simulink model "gm_sampleModel1739_2_sub"  (R2023a)
settings: Solver=VariableStepAuto  StartTime=0.0  StopTime=10.0  RelTol=1e-3
libraries: hdlsllib x2, simulink x1
settings Model: Creator=user1  LastModifiedBy=user1
settings OptimizationCC: BlockReduction=off  ConditionallyExecuteInputs=off
settings DebuggingCC: InheritedTsInSrcMsg=none

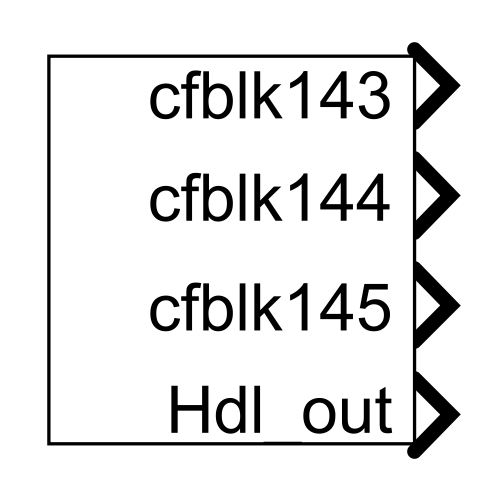
[thumbnail: Simulink's stored preview of the top-level diagram]
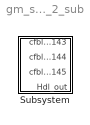
== system gm_sampleModel1739_2_sub ==
  Subsystem : Subsystem

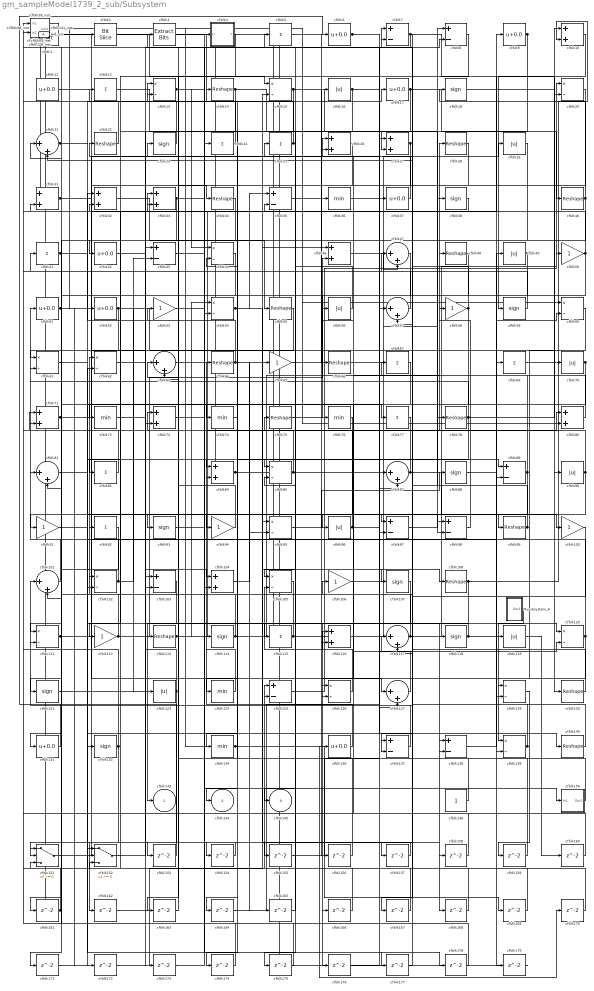
== system gm_sampleModel1739_2_sub/Subsystem ==
  Mysubsystem_6 : Subsystem
  cfblk1 : hdlsllib/Logic and Bit Operations/Bit Shift  mode=Shift Left Logical  N=0
  cfblk{10,26..27,31..33,46,71,73,80,84,104,116} (13 alike) : Sum  OutDataTypeStr=uint8
  cfblk{50,53,58,65,91,94,100,106,112} (9 alike) : Gain  OutDataTypeStr=uint8
  cfblk{21,47,57,63,81,87,101,117,127} (9 alike) : Sum  Inputs=|++  OutDataTypeStr=uint8
  cfblk{13,15,20,44,54,60..62,85,95,102,105,111,120,126,129,139} (17 alike) : Product  Inputs=*/  OutDataTypeStr=uint8  RndMeth=Zero  SaturateOnIntegerOverflow=on
  cfblk{7..8,35,43,89,97..98,103,125,137..138} (11 alike) : Sum  Inputs=+-  OutDataTypeStr=uint8
  cfblk{18,23,38,59,88,93,107,114,118,121,132} (11 alike) : Signum
  cfblk{14,22,28,34,40,48,55,64,66,75,78,99,108,113,130,140} (16 alike) : Reshape
  cfblk109_inst : Subsystem
  cfblk{6,9,11,17,37,42,51..52,131,136} (10 alike) : Bias  Bias=0.0  SaturateOnIntegerOverflow=off
  cfblk110_inst : Subsystem
  cfblk{5,12,24..25,41,67,69,77,82,92,115} (11 alike) : Sum  Inputs=+  OutDataTypeStr=uint8
  cfblk{16,29,49,56,70,90,96,119,123} (9 alike) : Abs  OutDataTypeStr=uint8  SaturateOnIntegerOverflow=off
  cfblk{36,72,74,76,124,134} (6 alike) : MinMax  OutDataTypeStr=uint8
  cfblk128_inst : Subsystem
  cfblk133_inst : Subsystem
  cfblk141_inst : Subsystem
  cfblk148 : Constant  OutDataTypeStr=uint8  SampleTime=-1
  cfblk150 : Subsystem
  cfblk151 : Switch  OutDataTypeStr=uint8  SaturateOnIntegerOverflow=off  InputSameDT=off
  cfblk152 : Switch  OutDataTypeStr=uint8  SaturateOnIntegerOverflow=off  InputSameDT=off
  cfblk{153..179} (27 alike) : Delay  SampleTime=1
  cfblk2 : hdlsllib/Logic and Bit Operations/Bit Slice  lidx=7  ridx=0
  cfblk3 : simulink/Logic and Bit Operations/Extract Bits  bitsToExtract=Upper half  numBits=8  bitIdxRange=[0 7]  outScalingMode=Preserve fixed-point scaling
      settings: LibrarySourceBlock=|
      | hdlsllib/Logic and Bit
      | Operations/Extract Bits
  cfblk39_inst : Subsystem
  cfblk4 : Subsystem  mask(Detect Rise Nonnegative){vinit=double(0), InputProcessing=Elements as channels (sample based), OutDataTypeStr=uint8}
      mask prompts: vinit "Simulink:masks:InitialCondition_MP"; InputProcessing "Simulink:masks:InputProcessing_MP"; OutDataTypeStr "Simulink:masks:OutputDataType_MP"
      mask help: Simulink:masks:DetectRiseNonnegative_MD
      mask init:
      | InputProcessing = 'Elements as channels (sample based)';
      | OutDataTypeStr = 'uint8';
      | vinit = double(0);
      mask TypeOptions InputProcessing: Simulink:masks:ColumnsAsChannelsFrameBased | Simulink:masks:ElementsAsChannelsSampleBased
      mask TypeOptions OutDataTypeStr: Simulink:masks:uint8 | Simulink:masks:boolean
      mask Display: fprintf('U >= 0\n&  NOT\nU/z >= 0')
  cfblk68_inst : Subsystem
  cfblk83_inst : Subsystem
  cfblk143 : Outport  OutDataTypeStr=uint8  SampleTime=1  VectorParamsAs1DForOutWhenUnconnected=off
  cfblk144 : Outport  Port=2  OutDataTypeStr=uint8  SampleTime=1  VectorParamsAs1DForOutWhenUnconnected=off
  cfblk145 : Outport  Port=3  OutDataTypeStr=uint8  SampleTime=1  VectorParamsAs1DForOutWhenUnconnected=off
  Hdl_out : Outport  Port=4  OutDataTypeStr=uint8  SampleTime=1
  wires:
  Mysubsystem_6/1(Out1) -> cfblk139/1
  cfblk1/1 -> cfblk34/1, cfblk127/1
  cfblk10/1 -> cfblk59/1
  cfblk100/1 -> cfblk125/1
  cfblk101/1 -> cfblk51/1
  cfblk102/1 -> cfblk81/1, cfblk43/2
  cfblk103/1 -> cfblk143/1
  cfblk104/1 -> cfblk65/1
  cfblk105/1 -> cfblk63/1
  cfblk106/1 -> cfblk29/1
  cfblk107/1 -> cfblk176/1
  cfblk108/1 -> cfblk10/2, cfblk168/1
  cfblk109_inst/1(out1) -> cfblk2/1
  cfblk11/1 -> cfblk77/1
  cfblk110_inst/1(out1) -> cfblk133_inst/2(in2), cfblk133_inst/1(in1), cfblk119/1
  cfblk111/1 -> cfblk35/2, cfblk23/1
  cfblk112/1 -> cfblk46/2, cfblk141_inst/1(in1)
  cfblk113/1 -> cfblk9/1, cfblk80/1, cfblk54/1
  cfblk114/1 -> cfblk71/2, cfblk28/1
  cfblk115/1 -> cfblk39_inst/1(in1), cfblk21/1
  cfblk116/1 -> cfblk48/1
  cfblk117/1 -> cfblk62/1, cfblk20/1
  cfblk118/1 -> cfblk113/1, cfblk60/2
  cfblk119/1 -> cfblk160/1
  cfblk12/1 -> cfblk98/1
  cfblk120/1 -> cfblk64/1, cfblk167/1, cfblk166/1
  cfblk121/1 -> cfblk103/2
  cfblk123/1 -> cfblk103/1, cfblk153/1
  cfblk124/1 -> cfblk84/2
  cfblk125/1 -> cfblk50/1
  cfblk126/1 -> cfblk105/2
  cfblk127/1 -> cfblk26/1
  cfblk128_inst/1(out1) -> cfblk87/1
  cfblk129/1 -> cfblk159/1
  cfblk13/1 -> cfblk54/2, cfblk44/1
  cfblk130/1 -> cfblk92/1
  cfblk131/1 -> cfblk6/1
  cfblk132/1 -> cfblk68_inst/1(in1), cfblk32/2, cfblk162/1
  cfblk133_inst/1(out1) -> cfblk60/1
  cfblk134/1 -> cfblk170/1, cfblk169/1
  cfblk136/1 -> cfblk114/1
  cfblk137/1 -> cfblk101/1
  cfblk138/1 -> cfblk69/1
  cfblk139/1 -> cfblk73/1, cfblk110_inst/2(in2), cfblk106/1
  cfblk14/1 -> cfblk63/2, cfblk27/2
  cfblk140/1 -> cfblk22/1
  cfblk141_inst/1(out1) -> cfblk31/1, cfblk136/1
  cfblk148/1 -> cfblk5/1
  cfblk15/1 -> cfblk78/1, cfblk73/2, cfblk57/1
  cfblk150/1(Out1) -> cfblk26/2
  cfblk151/1 -> cfblk49/1
  cfblk152/1 -> cfblk7/1
  cfblk153/1 -> cfblk109_inst/2(in2)
  cfblk154/1 -> cfblk152/2
  cfblk155/1 -> cfblk87/2
  cfblk156/1 -> cfblk44/2
  cfblk157/1 -> cfblk151/2
  cfblk158/1 -> cfblk83_inst/2(in2)
  cfblk159/1 -> cfblk13/1
  cfblk16/1 -> cfblk37/1, cfblk174/1
  cfblk160/1 -> cfblk116/1
  cfblk161/1 -> cfblk39_inst/2(in2), Hdl_out/1
  cfblk162/1 -> cfblk15/2
  cfblk163/1 -> cfblk33/1
  cfblk164/1 -> cfblk120/2
  cfblk165/1 -> cfblk85/2
  cfblk166/1 -> cfblk152/3
  cfblk167/1 -> cfblk125/2
  cfblk168/1 -> cfblk102/1
  cfblk169/1 -> cfblk57/2
  cfblk17/1 -> cfblk40/1, cfblk105/1
  cfblk170/1 -> cfblk151/3
  cfblk171/1 -> cfblk62/2
  cfblk172/1 -> cfblk95/1
  cfblk173/1 -> cfblk7/2
  cfblk174/1 -> cfblk31/2
  cfblk175/1 -> cfblk111/2
  cfblk176/1 -> cfblk97/2
  cfblk177/1 -> cfblk117/1
  cfblk178/1 -> cfblk128_inst/2(in2)
  cfblk179/1 -> cfblk1/1
  cfblk18/1 -> cfblk130/1
  cfblk2/1 -> cfblk15/1
  cfblk20/1 -> cfblk144/1
  cfblk21/1 -> cfblk17/1, cfblk120/1
  cfblk22/1 -> cfblk109_inst/1(in1)
  cfblk23/1 -> cfblk128_inst/1(in1)
  cfblk24/1 -> cfblk4/1(U)
  cfblk25/1 -> cfblk175/1, cfblk12/1
  cfblk26/1 -> cfblk134/1
  cfblk27/1 -> cfblk164/1, cfblk163/1
  cfblk28/1 -> cfblk157/1
  cfblk29/1 -> cfblk42/1
  cfblk3/1 -> cfblk24/1
  cfblk31/1 -> cfblk84/1, cfblk27/1
  cfblk32/1 -> cfblk55/1
  cfblk33/1 -> cfblk96/1, cfblk102/2
  cfblk34/1 -> cfblk111/1
  cfblk35/1 -> cfblk16/1
  cfblk36/1 -> cfblk138/2
  cfblk37/1 -> cfblk3/1
  cfblk38/1 -> cfblk33/2
  cfblk39_inst/1(out1) -> cfblk11/1
  cfblk4/1(Y) -> cfblk93/1
  cfblk40/1 -> cfblk18/1, cfblk171/1
  cfblk41/1 -> cfblk140/1, cfblk178/1
  cfblk42/1 -> cfblk118/1
  cfblk43/1 -> cfblk104/2
  cfblk44/1 -> cfblk91/1
  cfblk46/1 -> cfblk47/2
  cfblk47/1 -> cfblk76/1
  cfblk48/1 -> cfblk115/1
  cfblk49/1 -> cfblk97/1, cfblk121/1
  cfblk5/1 -> cfblk137/2
  cfblk50/1 -> cfblk141_inst/2(in2), cfblk112/1
  cfblk51/1 -> cfblk132/1, cfblk173/1, cfblk172/1
  cfblk52/1 -> cfblk90/1, cfblk81/2, cfblk123/1
  cfblk53/1 -> cfblk177/1
  cfblk54/1 -> cfblk46/1, cfblk35/1, cfblk126/2
  cfblk55/1 -> cfblk61/1
  cfblk56/1 -> cfblk25/1
  cfblk57/1 -> cfblk83_inst/1(in1)
  cfblk58/1 -> cfblk21/2, cfblk126/1
  cfblk59/1 -> cfblk47/1
  cfblk6/1 -> cfblk127/2, cfblk108/1
  cfblk60/1 -> cfblk129/1
  cfblk61/1 -> cfblk74/1
  cfblk62/1 -> cfblk99/1
  cfblk63/1 -> cfblk89/1
  cfblk64/1 -> cfblk32/1, cfblk165/1
  cfblk65/1 -> cfblk36/1
  cfblk66/1 -> cfblk38/1
  cfblk67/1 -> cfblk154/1
  cfblk68_inst/1(out1) -> cfblk66/1
  cfblk69/1 -> cfblk10/1
  cfblk7/1 -> cfblk70/1, cfblk68_inst/2(in2), cfblk117/2, cfblk129/2
  cfblk70/1 -> cfblk101/2, cfblk124/1
  cfblk71/1 -> cfblk89/2, cfblk156/1
  cfblk72/1 -> cfblk104/1
  cfblk73/1 -> cfblk138/1
  cfblk74/1 -> cfblk14/1
  cfblk75/1 -> cfblk116/2
  cfblk76/1 -> cfblk161/1
  cfblk77/1 -> cfblk94/1
  cfblk78/1 -> cfblk61/2, cfblk20/2, cfblk145/1
  cfblk8/1 -> cfblk82/1
  cfblk80/1 -> cfblk56/1
  cfblk81/1 -> cfblk98/2
  cfblk82/1 -> cfblk110_inst/1(in1)
  cfblk83_inst/1(out1) -> cfblk80/2, cfblk52/1
  cfblk84/1 -> cfblk107/1, cfblk95/2, cfblk158/1
  cfblk85/1 -> cfblk75/1, cfblk43/1
  cfblk87/1 -> cfblk85/1, cfblk179/1
  cfblk88/1 -> cfblk139/2
  cfblk89/1 -> cfblk155/1, cfblk67/1
  cfblk9/1 -> cfblk137/1, cfblk72/1
  cfblk90/1 -> cfblk151/1, cfblk53/1
  cfblk91/1 -> cfblk152/1
  cfblk92/1 -> cfblk131/1
  cfblk93/1 -> cfblk150/1(In1)
  cfblk94/1 -> cfblk13/2
  cfblk95/1 -> cfblk88/1
  cfblk96/1 -> cfblk8/2, cfblk71/1
  cfblk97/1 -> cfblk100/1
  cfblk98/1 -> cfblk58/1
  cfblk99/1 -> cfblk8/1, cfblk41/1

== system gm_sampleModel1739_2_sub/Subsystem/Mysubsystem_6 ==
  cfblk149 : Subsystem  mask(Counter Limited){uplimit=double(7), tsamp=double(-1)}
      mask prompts: uplimit "Simulink:masks:UpperLimit_MP"; tsamp "Simulink:masks:SampleTime_MP"
      mask help: Simulink:masks:CounterLimited_MD
      mask init:
      | nbits = double(8);
      | tsamp = double(-1);
      | uplimit = double(7);
  cfblk79 : Signum
  Out1 : Outport  SampleTime=1
  wires:
  cfblk149/1(y) -> cfblk79/1
  cfblk79/1 -> Out1/1

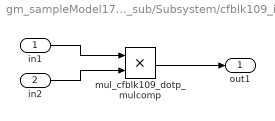
== system gm_sampleModel1739_2_sub/Subsystem/cfblk109_inst ==
  in1 : Inport  OutDataTypeStr=uint8  SampleTime=1
  in2 : Inport  Port=2  OutDataTypeStr=uint8  SampleTime=1
  mul_cfblk109_dotp_mulcomp : Product  Inputs=**  OutDataTypeStr=uint8  SampleTime=1
  out1 : Outport  OutDataTypeStr=uint8  SampleTime=1
  wires:
  in1/1 -> mul_cfblk109_dotp_mulcomp/1
  in2/1 -> mul_cfblk109_dotp_mulcomp/2
  mul_cfblk109_dotp_mulcomp/1 -> out1/1

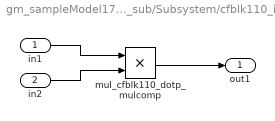
== system gm_sampleModel1739_2_sub/Subsystem/cfblk110_inst ==
  in1 : Inport  OutDataTypeStr=uint8  SampleTime=1
  in2 : Inport  Port=2  OutDataTypeStr=uint8  SampleTime=1
  mul_cfblk110_dotp_mulcomp : Product  Inputs=**  OutDataTypeStr=uint8  SampleTime=1
  out1 : Outport  OutDataTypeStr=uint8  SampleTime=1
  wires:
  in1/1 -> mul_cfblk110_dotp_mulcomp/1
  in2/1 -> mul_cfblk110_dotp_mulcomp/2
  mul_cfblk110_dotp_mulcomp/1 -> out1/1

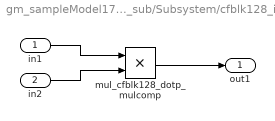
== system gm_sampleModel1739_2_sub/Subsystem/cfblk128_inst ==
  in1 : Inport  OutDataTypeStr=uint8  SampleTime=1
  in2 : Inport  Port=2  OutDataTypeStr=uint8  SampleTime=1
  mul_cfblk128_dotp_mulcomp : Product  Inputs=**  OutDataTypeStr=uint8  SampleTime=1
  out1 : Outport  OutDataTypeStr=uint8  SampleTime=1
  wires:
  in1/1 -> mul_cfblk128_dotp_mulcomp/1
  in2/1 -> mul_cfblk128_dotp_mulcomp/2
  mul_cfblk128_dotp_mulcomp/1 -> out1/1

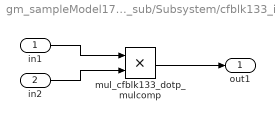
== system gm_sampleModel1739_2_sub/Subsystem/cfblk133_inst ==
  in1 : Inport  OutDataTypeStr=uint8  SampleTime=1
  in2 : Inport  Port=2  OutDataTypeStr=uint8  SampleTime=1
  mul_cfblk133_dotp_mulcomp : Product  Inputs=**  OutDataTypeStr=uint8  SampleTime=1
  out1 : Outport  OutDataTypeStr=uint8  SampleTime=1
  wires:
  in1/1 -> mul_cfblk133_dotp_mulcomp/1
  in2/1 -> mul_cfblk133_dotp_mulcomp/2
  mul_cfblk133_dotp_mulcomp/1 -> out1/1

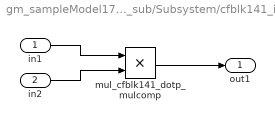
== system gm_sampleModel1739_2_sub/Subsystem/cfblk141_inst ==
  in1 : Inport  OutDataTypeStr=uint8  SampleTime=1
  in2 : Inport  Port=2  OutDataTypeStr=uint8  SampleTime=1
  mul_cfblk141_dotp_mulcomp : Product  Inputs=**  OutDataTypeStr=uint8  SampleTime=1
  out1 : Outport  OutDataTypeStr=uint8  SampleTime=1
  wires:
  in1/1 -> mul_cfblk141_dotp_mulcomp/1
  in2/1 -> mul_cfblk141_dotp_mulcomp/2
  mul_cfblk141_dotp_mulcomp/1 -> out1/1

== system gm_sampleModel1739_2_sub/Subsystem/cfblk150 ==
  In1 : Inport  OutDataTypeStr=uint8  PortDimensions=1  SampleTime=1
  Out1 : Outport  SampleTime=1
  wires:
  In1/1 -> Out1/1

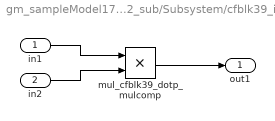
== system gm_sampleModel1739_2_sub/Subsystem/cfblk39_inst ==
  in1 : Inport  OutDataTypeStr=uint8  SampleTime=1
  in2 : Inport  Port=2  OutDataTypeStr=uint8  SampleTime=1
  mul_cfblk39_dotp_mulcomp : Product  Inputs=**  OutDataTypeStr=uint8  SampleTime=1
  out1 : Outport  OutDataTypeStr=uint8  SampleTime=1
  wires:
  in1/1 -> mul_cfblk39_dotp_mulcomp/1
  in2/1 -> mul_cfblk39_dotp_mulcomp/2
  mul_cfblk39_dotp_mulcomp/1 -> out1/1

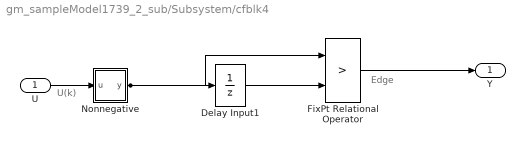
== system gm_sampleModel1739_2_sub/Subsystem/cfblk4 ==
  note: U(k)
  note: Edge
  U : Inport  OutDataTypeStr=uint8  SampleTime=1
  Delay Input1 : UnitDelay  Description=Store in Global RAM  DisableCoverage=on  InitialCondition=vinit  SampleTime=-1  HasFrameUpgradeWarning=on
  FixPt Relational Operator : RelationalOperator  Operator=>  OutDataTypeStr=fixdt(0, 8)  ZeroCross=off  InputSameDT=off
  Nonnegative : Subsystem  mask(Compare To Zero){relop=>=, OutDataTypeStr=boolean, ZeroCross=off}
      mask prompts: relop "Simulink:masks:Operator_MP"; OutDataTypeStr "Simulink:masks:OutputDataType_MP"; ZeroCross "Simulink:masks:EnableZerocrossingDetection_MP"
      mask help: Simulink:masks:CompareToZero_MD
      mask init:
      | OutDataTypeStr = 'boolean';
      | ZeroCross = 'off';
      | blkName = 'sampleModel1739_2_sub/Subsystem/cfblk4/Nonnegative';
      | relop = '>=';
      | setValue = 'boolean';
      mask TypeOptions relop: == | ~= | < | <= | >= | >
      mask TypeOptions OutDataTypeStr: Simulink:masks:uint8 | Simulink:masks:boolean
      mask Callback ZeroCross: sl('zeroCrossEnable', gcbh);
      mask Display: disp([relop,' 0'])
  Y : Outport  SampleTime=1
  wires:
  U/1 -> Nonnegative/1(u)
  Delay Input1/1 -> FixPt Relational Operator/2
  FixPt Relational Operator/1 -> Y/1
  Nonnegative/1(y) -> FixPt Relational Operator/1, Delay Input1/1

== system gm_sampleModel1739_2_sub/Subsystem/cfblk68_inst ==
  in1 : Inport  OutDataTypeStr=uint8  SampleTime=1
  in2 : Inport  Port=2  OutDataTypeStr=uint8  SampleTime=1
  mul_cfblk68_dotp_mulcomp : Product  Inputs=**  OutDataTypeStr=uint8  SampleTime=1
  out1 : Outport  OutDataTypeStr=uint8  SampleTime=1
  wires:
  in1/1 -> mul_cfblk68_dotp_mulcomp/1
  in2/1 -> mul_cfblk68_dotp_mulcomp/2
  mul_cfblk68_dotp_mulcomp/1 -> out1/1

== system gm_sampleModel1739_2_sub/Subsystem/cfblk83_inst ==
  in1 : Inport  OutDataTypeStr=uint8  SampleTime=1
  in2 : Inport  Port=2  OutDataTypeStr=uint8  SampleTime=1
  mul_cfblk83_dotp_mulcomp : Product  Inputs=**  OutDataTypeStr=uint8  SampleTime=1
  out1 : Outport  OutDataTypeStr=uint8  SampleTime=1
  wires:
  in1/1 -> mul_cfblk83_dotp_mulcomp/1
  in2/1 -> mul_cfblk83_dotp_mulcomp/2
  mul_cfblk83_dotp_mulcomp/1 -> out1/1

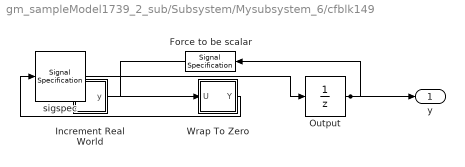
== system gm_sampleModel1739_2_sub/Subsystem/Mysubsystem_6/cfblk149 ==
  Force to be scalar : SignalSpecification  DisableCoverage=on  Dimensions=1
  Increment Real World : Subsystem  mask(Real World Value Increment){}
      mask help: Simulink:masks:RealWorldValueIncrement_MD
      mask Display: disp('V++')
  Output : UnitDelay  InitialCondition=0.0  SampleTime=tsamp  HasFrameUpgradeWarning=on
  Wrap To Zero : Subsystem  mask(Wrap To Zero){Threshold=double(7)}
      mask prompts: Threshold "Simulink:masks:Threshold_MP"
      mask help: Simulink:masks:WrapToZero_MD
  sigspec : SignalSpecification  OutDataTypeStr=uint8  Dimensions=1
  y : Outport  SampleTime=1
  wires:
  Force to be scalar/1 -> Increment Real World/1(u)
  Increment Real World/1(y) -> Wrap To Zero/1(U)
  Output/1 -> Force to be scalar/1, y/1
  Wrap To Zero/1(Y) -> sigspec/1
  sigspec/1 -> Output/1

== system gm_sampleModel1739_2_sub/Subsystem/cfblk4/Nonnegative ==
  u : Inport  OutDataTypeStr=uint8  SampleTime=1
  Compare : RelationalOperator  OutDataTypeStr=boolean  ZeroCross=off
  Constant : Constant  DisableCoverage=on  Value=0  OutDataTypeStr=Inherit: Inherit via back propagation  SampleTime=-1  PreserveConstantTs=on
  y : Outport  SampleTime=1
  wires:
  u/1 -> Compare/1
  Compare/1 -> y/1
  Constant/1 -> Compare/2

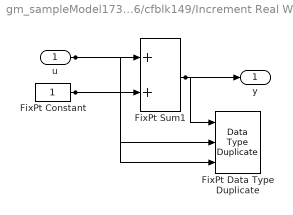
== system gm_sampleModel1739_2_sub/Subsystem/Mysubsystem_6/cfblk149/Increment Real World ==
  u : Inport  OutDataTypeStr=uint8  SampleTime=1
  FixPt Constant : Constant  DisableCoverage=on  OutDataTypeStr=Inherit: Inherit via back propagation  SampleTime=-1
  FixPt Data Type Duplicate : DataTypeDuplicate  DisableCoverage=on  NumInputPorts=3
  FixPt Sum1 : Sum  InputSameDT=on  OutDataTypeStr=Inherit: Inherit via back propagation  LockScale=on
  y : Outport  SampleTime=1
  wires:
  u/1 -> FixPt Sum1/1, FixPt Data Type Duplicate/2
  FixPt Constant/1 -> FixPt Sum1/2, FixPt Data Type Duplicate/3
  FixPt Sum1/1 -> FixPt Data Type Duplicate/1, y/1

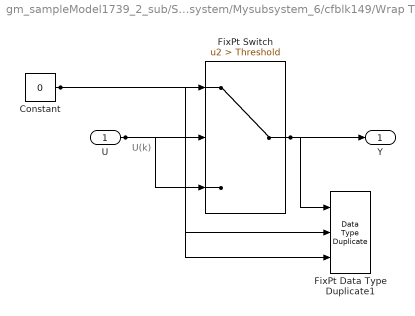
== system gm_sampleModel1739_2_sub/Subsystem/Mysubsystem_6/cfblk149/Wrap To Zero ==
  note: U(k)
  U : Inport  OutDataTypeStr=uint8  SampleTime=1
  Constant : Constant  DisableCoverage=on  Value=0  OutDataTypeStr=Inherit: Inherit via back propagation  SampleTime=-1
  FixPt Data Type Duplicate1 : DataTypeDuplicate  DisableCoverage=on  NumInputPorts=3
  FixPt Switch : Switch  Criteria=u2 > Threshold  Threshold=Threshold  OutDataTypeStr=Inherit: Inherit via back propagation  ZeroCross=off  SaturateOnIntegerOverflow=off  InputSameDT=off
  Y : Outport  SampleTime=1
  wires:
  U/1 -> FixPt Switch/3, FixPt Switch/2, FixPt Data Type Duplicate1/2
  Constant/1 -> FixPt Switch/1, FixPt Data Type Duplicate1/3
  FixPt Switch/1 -> FixPt Data Type Duplicate1/1, Y/1
